simulink model "Regenerative_Brakes_PMSM_simscape"  (R2025b)
settings: Solver=ode23t  StartTime=0.0  StopTime=2.5  RelTol=1e-3  EnableMultiTasking=on
undefined symbols (not defined in the file): PermanentMagnetSynchrono_class, sigbuilder_block, Three_PhaseFault_class, UniversalBridge_class
libraries: nesl_utility x15, fl_lib x12, ee_lib x7, eeTransforms x2
settings Model: Creator=noname
settings SolverCC: AlgebraicLoopSolver=TrustRegion
settings DataIOCC: LimitDataPoints=on  SaveFormat=Array  ReturnWorkspaceOutputs=off
settings OptimizationCC: LifeSpan=inf
settings DebuggingCC: SaveWithParameterizedLinksMsg=none  UnderspecifiedInitializationDetection=Classic  MergeDetectMultiDrivingBlocksExec=none  SolverPrmCheckMsg=warning  UnconnectedInputMsg=warning  UnconnectedOutputMsg=warning  UnconnectedLineMsg=warning  StateNameClashWarn=warning  SFUnexpectedBacktrackingDiag=warning  SFNoUnconditionalDefaultTransitionDiag=warning  SFExecutionAtInitializationDiag=none  ArithmeticOperatorsInVariantConditions=warning
settings HardwareCC: ProdBitPerPointer=32.0  ProdBitPerSizeT=32.0  ProdBitPerPtrDiffT=32.0  ProdLargestAtomicFloat=None  ProdIntDivRoundTo=Undefined  ProdEndianess=Unspecified  ProdWordSize=32.0  ProdHWDeviceType=32-bit Generic
settings ModelReferenceCC: EnableRefExpFcnMdlSchedulingChecks=on  PropagateSignalLabelsOutOfModel=off
settings SFSimCC: SimUseLocalCustomCode=off  CustomCodeUndefinedFunction=UseInterfaceOnly
settings RTWCC: RTWUseLocalCustomCode=off  GPUComputeCapability=3.5  DLArmComputeVersion=19.05
settings CodeAppCC: StateflowObjectComments=on
settings GRTTargetCC: TargetLangStandard=C89/C90 (ANSI)
settings ConfigComp: CovMetricSettings=dw  CovSaveCumulativeToWorkspaceVar=on  CovSaveSingleToWorkspaceVar=on  CovExternalEMLEnable=off
settings SimscapeCC: SimscapeNormalizeSystem=off

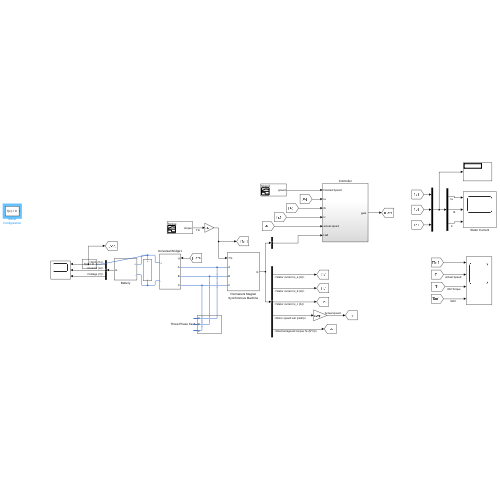
[thumbnail: Simulink's stored preview of the top-level diagram]
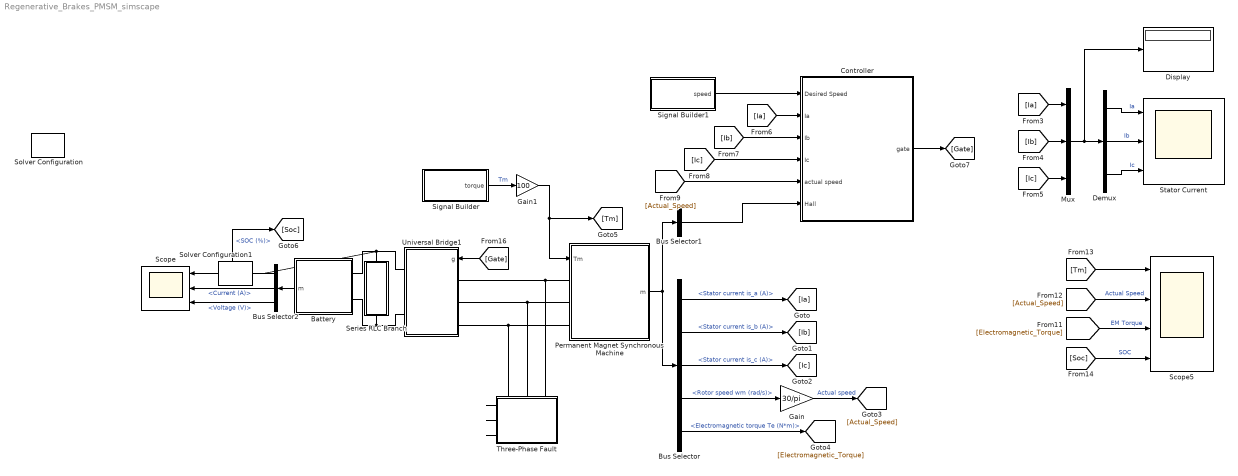
== system Regenerative_Brakes_PMSM_simscape ==
  Battery : Subsystem
      settings: OpenFcn=elec.conv.unmask(gcb);
  Bus Selector : BusSelector  OutputSignals=Stator current is_a (A),Stator current is_b (A),Stator current is_c (A),Rotor speed wm (rad/s),Electromagnetic torque Te (N*m)
  Bus Selector1 : BusSelector  OutputSignals=Hall effect signal h_a,Hall effect signal h_b,Hall effect signal h_c  OutputAsBus=on
  Bus Selector2 : BusSelector  OutputSignals=SOC (%),Current (A),Voltage (V)
  Controller : Subsystem
  Demux : Demux  Outputs=3
  Display : Display
  Gain : Gain  Gain=30/pi
  Gain1 : Gain  Gain=100
  Mux : Mux  Inputs=3
  Permanent Magnet Synchronous Machine : Subsystem
      settings: OpenFcn=elec.conv.unmask(gcb);
  Scope : Scope  NumInputPorts=3
      settings: ActiveDisplayYMinimum=79.5644  ActiveDisplayYMaximum=80.0484
  Scope5 : Scope  NumInputPorts=4
      settings: ActiveDisplayYMinimum=-400  ActiveDisplayYMaximum=600  DataLoggingVariableName=ScopeData13
  Series RLC Branch : Subsystem
      settings: OpenFcn=elec.conv.unmask(gcb);
  Signal Builder : Subsystem  Tag=STV Subsys  LoadFcn=sigbuilder_block('load');  StartFcn=sigbuilder_block('start');  StopFcn=sigbuilder_block('stop');  ClipboardFcn=sigbuilder_block('clipboard');  mask(Sigbuilder block){tuvar=[0:10]}
      mask help: Simulink:masks:SigbuilderBlock_MD
      mask init:
      | if ~strcmp(get_param(bdroot(gcbh),'SimulationStatus'),'stopped') tuvar = sigbuilder_block('maskInit'); end
      settings: CopyFcn=sigbuilder_block('copy');  DeleteFcn=sigbuilder_block('delete');  ModelCloseFcn=sigbuilder_block('modelClose');  PreSaveFcn=sigbuilder_block('preSave');  PauseFcn=sigbuilder_block('pause');  ContinueFcn=sigbuilder_block('continue');  NameChangeFcn=sigbuilder_block('namechange');  OpenFcn=sigbuilder_block('open',[437.25 183.75 550.5 395.25 ]);  CloseFcn=sigbuilder_block('close');
      mask Display: plot(0, 0, 100, 100,[2, 2, 32, 32, 2], [68, 8, 8, 68, 68],[32, 2], [38, 38], [32, 19, 2],[53, 60, 44], [32, 17, 17, 2],[16, 16, 31, 31]);txt = getActiveGroup(gcbh);text(2, 100, txt,'verticalAlignment', 'top');
  Signal Builder1 : Subsystem  Tag=STV Subsys  LoadFcn=sigbuilder_block('load');  StartFcn=sigbuilder_block('start');  StopFcn=sigbuilder_block('stop');  ClipboardFcn=sigbuilder_block('clipboard');  mask(Sigbuilder block){tuvar=[0:10]}
      mask help: Simulink:masks:SigbuilderBlock_MD
      mask init:
      | if ~strcmp(get_param(bdroot(gcbh),'SimulationStatus'),'stopped') tuvar = sigbuilder_block('maskInit'); end
      settings: CopyFcn=sigbuilder_block('copy');  DeleteFcn=sigbuilder_block('delete');  ModelCloseFcn=sigbuilder_block('modelClose');  PreSaveFcn=sigbuilder_block('preSave');  PauseFcn=sigbuilder_block('pause');  ContinueFcn=sigbuilder_block('continue');  NameChangeFcn=sigbuilder_block('namechange');  OpenFcn=sigbuilder_block('open',[6.75 6.75 1138.5 568.5 ]);  CloseFcn=sigbuilder_block('close');
      mask Display: plot(0, 0, 100, 100,[2, 2, 32, 32, 2], [68, 8, 8, 68, 68],[32, 2], [38, 38], [32, 19, 2],[53, 60, 44], [32, 17, 17, 2],[16, 16, 31, 31]);txt = getActiveGroup(gcbh);text(2, 100, txt,'verticalAlignment', 'top');
  Solver Configuration : nesl_utility/Solver Configuration  PhysicalDomain=network_engine_domain  SubClassName=solver  LeftPortType=input  RightPortType=generic  Tones=[]  Harmonics=[]  SimulateNoise=off  Profile=off  UseLocalSampling=off  EnableSwitchedLinearOptims=on  FrequencyDomain=off  UseCCode=off  RelTol=0.001  AbsTol=0.001  MinStep=1e-09  ToWorkspace=off  RevertToSquareIcSolve=off  NumHomotopyIterations=100  PhasorMode=off  PhasorModeNumHarmonics=1  ConsistencySolver=NEWTON_XTOL_AFTER_FTOL  IndexReductionMethod=DerivativeReplacement  DoDC=off  ResidualTolerance=1e-09  ConsistencyTolSource=GLOBAL  ConsistencyAbsTol=0.001  ConsistencyRelTol=0.001  ConsistencyTolFactor=0.001  UseLocalSolver=off  LocalSolverChoice=NE_BACKWARD_EULER_ADVANCER  ResolveIndetEquations=on  FunctionEvalNumThread=1  LocalSolverSampleTime=0.001  DoFixedCost=off  MaxNonlinIter=3  MaxModeIter=2  ComputeImpulses=off  ImpulseIterations=2  LinearAlgebra=auto  LinearAlgebraNumThread=0  EquationFormulation=NE_TIME_EF  DelaysMemoryBudget=1024  AutomaticFiltering=on  FilteringTimeConstant=0.001  PartitionStorageMethod=AS_NEEDED  PartitionMemoryBudget=1024  PartitionMethod=ROBUST  MultibodyUseLocalSolver=off  MultibodyLocalSolverChoice=ODE1  MultibodyLocalSolverSampleTime=0.001
  Solver Configuration1 : nesl_utility/Solver Configuration  PhysicalDomain=network_engine_domain  SubClassName=solver  LeftPortType=input  RightPortType=generic  Tones=[]  Harmonics=[]  SimulateNoise=off  Profile=off  UseLocalSampling=off  EnableSwitchedLinearOptims=on  FrequencyDomain=off  UseCCode=off  RelTol=0.001  AbsTol=0.001  MinStep=1e-09  ToWorkspace=off  RevertToSquareIcSolve=off  NumHomotopyIterations=100  PhasorMode=off  PhasorModeNumHarmonics=1  ConsistencySolver=NEWTON_XTOL_AFTER_FTOL  IndexReductionMethod=DerivativeReplacement  DoDC=off  ResidualTolerance=1e-09  ConsistencyTolSource=GLOBAL  ConsistencyAbsTol=0.001  ConsistencyRelTol=0.001  ConsistencyTolFactor=0.001  UseLocalSolver=off  LocalSolverChoice=NE_BACKWARD_EULER_ADVANCER  ResolveIndetEquations=on  FunctionEvalNumThread=1  LocalSolverSampleTime=0.001  DoFixedCost=off  MaxNonlinIter=3  MaxModeIter=2  ComputeImpulses=off  ImpulseIterations=2  LinearAlgebra=auto  LinearAlgebraNumThread=0  EquationFormulation=NE_TIME_EF  DelaysMemoryBudget=1024  AutomaticFiltering=on  FilteringTimeConstant=0.001  PartitionStorageMethod=AS_NEEDED  PartitionMemoryBudget=1024  PartitionMethod=ROBUST  MultibodyUseLocalSolver=off  MultibodyLocalSolverChoice=ODE1  MultibodyLocalSolverSampleTime=0.001
  Stator Current : Scope  NumInputPorts=3
      settings: ActiveDisplayYMinimum=-124.07803  ActiveDisplayYMaximum=125.94528
  Three-Phase Fault : Subsystem
      settings: OpenFcn=elec.conv.unmask(gcb);
  Universal Bridge1 : Subsystem
      settings: OpenFcn=elec.conv.unmask(gcb);
  wires:
  Permanent Magnet Synchronous Machine/1(m) -> Bus Selector/1, Bus Selector1/1
  Bus Selector/1 -> [Ia]  "<Stator current is_a (A)>"
  Bus Selector/2 -> [Ib]  "<Stator current is_b (A)>"
  Bus Selector/3 -> [Ic]  "<Stator current is_c (A)>"
  Bus Selector/4 -> Gain/1  "<Rotor speed wm (rad/s)>"
  Bus Selector1/1 -> Controller/6("Hall ")
  Gain/1 -> [Actual_Speed]  "Actual speed"
  Controller/1("gate ") -> [Gate]
  Battery/1(m) -> Bus Selector2/1
  Bus Selector2/1 -> Scope/1, [Soc]  "<SOC (%)>"
  Bus Selector2/2 -> Scope/2  "<Current (A)>"
  Bus Selector2/3 -> Scope/3  "<Voltage (V)>"
  Mux/1 -> Display/1, Demux/1
  Signal Builder/1(torque) -> Gain1/1  "Tm"
  Bus Selector/5 -> [Electromagnetic_Torque]  "<Electromagnetic torque Te (N*m)>"
  [Ia] -> Mux/1
  [Ib] -> Mux/2
  [Ic] -> Mux/3
  [Ia] -> Controller/2(Ia)
  [Ib] -> Controller/3(Ib)
  [Ic] -> Controller/4(Ic)
  [Actual_Speed] -> Controller/5(actual speed)
  [Actual_Speed] -> Scope5/2  "Actual Speed"
  [Tm] -> Scope5/1
  [Soc] -> Scope5/4  "SOC"
  [Gate] -> Universal Bridge1/1(g)
  Signal Builder1/1(speed) -> Controller/1(Desired Speed)
  Demux/1 -> Stator Current/1  "Ia"
  Demux/2 -> Stator Current/2  "Ib"
  Demux/3 -> Stator Current/3  "Ic"
  [Electromagnetic_Torque] -> Scope5/3  "EM Torque"
  Gain1/1 -> Permanent Magnet Synchronous Machine/1(Tm), [Tm]
  connections:
  Universal Bridge1/LConn1 -- Three-Phase Fault/LConn1 -- Permanent Magnet Synchronous Machine/LConn1
  Permanent Magnet Synchronous Machine/LConn2 -- Universal Bridge1/LConn2 -- Three-Phase Fault/LConn2
  Universal Bridge1/LConn3 -- Three-Phase Fault/LConn3 -- Permanent Magnet Synchronous Machine/LConn3
  Series RLC Branch/LConn1 -- Universal Bridge1/RConn1 -- Battery/LConn1 -- Solver Configuration1/RConn1
  Series RLC Branch/RConn1 -- Battery/LConn2 -- Universal Bridge1/RConn2

== system Regenerative_Brakes_PMSM_simscape/Battery ==
  + : PMIOPort  Side=Left
  - : PMIOPort  Port=2  Side=Left
  m : Outport  VectorParamsAs1DForOutWhenUnconnected=off

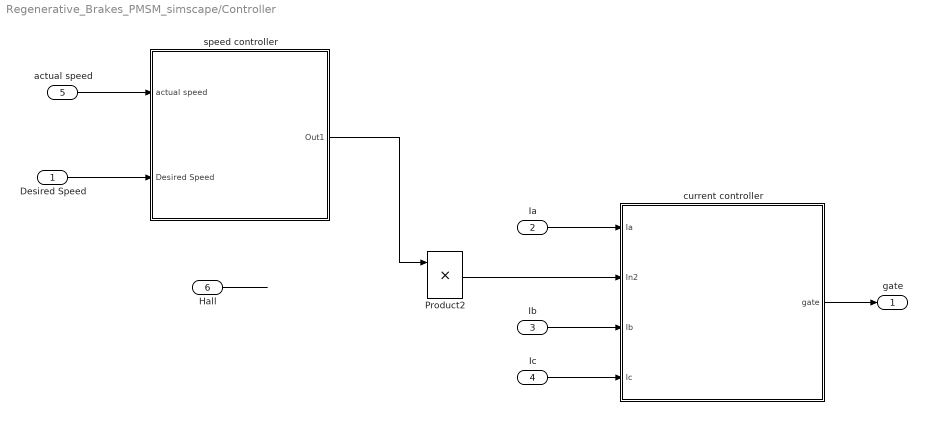
== system Regenerative_Brakes_PMSM_simscape/Controller ==
  Desired Speed : Inport
  Ia : Inport  Port=2
  Ib : Inport  Port=3
  Ic : Inport  Port=4
  actual speed : Inport  Port=5
  "Hall " : Inport  Port=6
  Product2 : Product  SaturateOnIntegerOverflow=on  OutDataTypeStr=Inherit: Same as first input
  current controller : Subsystem
  speed controller : Subsystem
  "gate " : Outport  VectorParamsAs1DForOutWhenUnconnected=off
  wires:
  "Hall "/1 -> ?
  ? -> Product2/2
  current controller/1("gate ") -> "gate "/1
  Ic/1 -> current controller/4(Ic)
  Ib/1 -> current controller/3(Ib)
  Ia/1 -> current controller/1(Ia)
  Product2/1 -> current controller/2(In2)
  actual speed/1 -> speed controller/1(actual speed)
  speed controller/1(Out1) -> Product2/1
  Desired Speed/1 -> speed controller/2(Desired Speed)

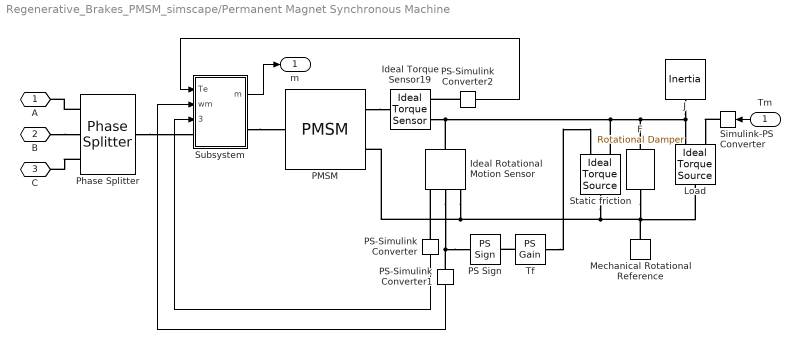
== system Regenerative_Brakes_PMSM_simscape/Permanent Magnet Synchronous Machine ==
  Tm : Inport
  F : fl_lib/Mechanical/Rotational Elements/Rotational Damper  D=0.000425 N*m/(rad/s)  w_specify=on  w_priority=High  w=0 rad/s  w_nominal_specify=off  w_nominal_value=1  w_nominal_unit=rad/s  t_specify=off  t_priority=None  t=0 N*m  t_nominal_specify=off  t_nominal_value=1  t_nominal_unit=N*m
  Ideal Rotational Motion Sensor : fl_lib/Mechanical/Mechanical Sensors/Ideal Rotational Motion Sensor  reference=foundation.enum.MeasurementReference.difference  acceleration_port=false  velocity_port=true  position_port=true  wrap_angle=simscape.enum.onoff.off  offset=0 deg
  Ideal Torque Sensor19 : fl_lib/Mechanical/Mechanical Sensors/Ideal Torque Sensor
  J : fl_lib/Mechanical/Rotational Elements/Inertia  inertia=0.003334 kg*m^2  num_ports=foundation.enum.numPorts2.one  w_specify=on  w_priority=High  w=0 rad/s  w_nominal_specify=off  w_nominal_value=1  w_nominal_unit=rad/s  t_specify=off  t_priority=None  t=0 N*m  t_nominal_specify=off  t_nominal_value=1  t_nominal_unit=N*m
  Load : fl_lib/Mechanical/Mechanical Sources/Ideal Torque Source
  Mechanical Rotational Reference : fl_lib/Mechanical/Rotational Elements/Mechanical Rotational Reference
  PMSM : ee_lib/Electromechanical/Permanent Magnet/PMSM  port_option=ee.enum.threePhasePort.composite  winding_type=ee.enum.statorconnection.wye  machine_param=ee.enum.pmsm.parameterization.constant  nPolePairs=4  pmflux_param=1  pm_flux_linkage=PermanentMagnetSynchrono_class('Torque Tm',[0.003334 0.000425 4 0],4,'Flux linkage established by magnets (V.s)',0.1821,132.1171,1.0926,'90 degrees behind phase A axis (modified Park)',[0 0 0 0],'Sinusoidal',120,'3',[0 0 0 0 0 0]).objParamMappingDerived.NewDerivedParam.pm_flux_linkage Wb  torque_constant=0.18 N*m/A  back_emf_constant=0.18 V/(rad/s)  stator_param=1  Ld=0.00153 H  Lq=0.00153 H  idVec=[-200, 0, 200] A  iqVec=[-200, 0, 200] A  LdMatrix=0.0002 * ones(3, 3) H  LqMatrix=0.0002 * ones(3, 3) H  PmMatrix=0.1 * ones(3, 3) Wb  ktMatrix=0.18 * ones(3, 3) N*m/A  keMatrix=0.18 * ones(3, 3) V/(rad/s)  L0=1e-09 H  Ls=0.0002 H  Lm=-0.00002 H  Ms=0.00002 H  Rs=0.129 Ohm  zero_sequence=0  axes_param=1  loss_param=ee.enum.ironloss.none  losses_oc=[0, 0, 0] W  losses_sc=[0, 0, 0] W  f_losses=60 Hz  Isc_losses=95 A  J=0 kg*m^2  lam=0 N*m/(rad/s)  i_d_specify=on  i_d_priority=High  i_d=PermanentMagnetSynchrono_class('Torque Tm',[0.003334 0.000425 4 0],4,'Flux linkage established by magnets (V.s)',0.1821,132.1171,1.0926,'90 degrees behind phase A axis (modified Park)',[0 0 0 0],'Sinusoidal',120,'3',[0 0 0 0 0 0]).objParamMappingDerived.NewDerivedParam.i_d A  i_d_nominal_specify=off  i_d_nominal_value=1  i_d_nominal_unit=A  i_q_specify=on  i_q_priority=High  i_q=PermanentMagnetSynchrono_class('Torque Tm',[0.003334 0.000425 4 0],4,'Flux linkage established by magnets (V.s)',0.1821,132.1171,1.0926,'90 degrees behind phase A axis (modified Park)',[0 0 0 0],'Sinusoidal',120,'3',[0 0 0 0 0 0]).objParamMappingDerived.NewDerivedParam.i_q A  i_q_nominal_specify=off  i_q_nominal_value=1  i_q_nominal_unit=A  torque_specify=off  torque_priority=None  torque=0 N*m  torque_nominal_specify=off  torque_nominal_value=1  torque_nominal_unit=N*m  angular_velocity_specify=on  angular_velocity_priority=High  angular_velocity=0 rad/s  angular_velocity_nominal_specify=off  angular_velocity_nominal_value=1  angular_velocity_nominal_unit=rpm  angular_position_specify=on  angular_position_priority=High  angular_position=0 deg  angular_position_nominal_specify=off  angular_position_nominal_value=1  angular_position_nominal_unit=deg  alpha=3.93e-3 1/K  alpha_flux=-0.001 1/K  Tmeas=298.15 K  stator_thermal_mass=100 J/K  rotor_thermal_mass=200 J/K  Rm_percent_rotor=90  Rd_percent_rotor=30  temperatureA_specify=off  temperatureA_priority=High  temperatureA=25 degC  temperatureA_nominal_specify=off  temperatureA_nominal_value=1  temperatureA_nominal_unit=degC  temperatureB_specify=off  temperatureB_priority=High  temperatureB=25 degC  temperatureB_nominal_specify=off  temperatureB_nominal_value=1  temperatureB_nominal_unit=degC  temperatureC_specify=off  temperatureC_priority=High  temperatureC=25 degC  temperatureC_nominal_specify=off  temperatureC_nominal_value=1  temperatureC_nominal_unit=degC  temperatureR_specify=off  temperatureR_priority=High  temperatureR=25 degC  temperatureR_nominal_specify=off  temperatureR_nominal_value=1  temperatureR_nominal_unit=degC
      settings: InternalSimscapePortConfiguration="{\"Bottom\":[],\"Left\":[{\"id\":\"N\",\"label\":\"~\",\"type\":\"foundation.electrical.three_phase\"}],\"Right\":[{\"id\":\"R\",\"label\":\"R\",\"type\":\"foundation.mechanical.rotational.rotational\"},{\"id\":\"C\",\"label\":\"C\",\"type\":\"foundation.mechanical.rotational.rotational\"}],\"Top\":[]}"
  PS Sign : fl_lib/Physical Signals/Nonlinear Operators/PS Sign
      settings: InternalSimscapePortConfiguration="{\"Bottom\":[],\"Left\":[{\"id\":\"I\",\"label\":\"\",\"type\":\"input\"}],\"Right\":[{\"id\":\"O\",\"label\":\"\",\"type\":\"output\"}],\"Top\":[]}"
  PS-Simulink Converter : nesl_utility/PS-Simulink Converter  PhysicalDomain=network_engine_domain  SubClassName=ps_output  LeftPortType=input  RightPortType=output  PseudoPeriodic=off  Frequencies=[]  VectorFormat=1-D array  Unit=1  AffineConversion=off
  PS-Simulink Converter1 : nesl_utility/PS-Simulink Converter  PhysicalDomain=network_engine_domain  SubClassName=ps_output  LeftPortType=input  RightPortType=output  PseudoPeriodic=off  Frequencies=[]  VectorFormat=1-D array  Unit=1  AffineConversion=off
  PS-Simulink Converter2 : nesl_utility/PS-Simulink Converter  PhysicalDomain=network_engine_domain  SubClassName=ps_output  LeftPortType=input  RightPortType=output  PseudoPeriodic=off  Frequencies=[]  VectorFormat=1-D array  Unit=1  AffineConversion=off
  Phase Splitter : ee_lib/Connectors & References/Phase Splitter
  Simulink-PS Converter : nesl_utility/Simulink-PS Converter  PhysicalDomain=network_engine_domain  SubClassName=ps_input  LeftPortType=input  RightPortType=output  PseudoPeriodic=off  Frequencies=[]  NoiseDistribution=none  NoiseParameters=[]  Unit=1  AffineConversion=off  FilteringAndDerivatives=provide  SimscapeFilterOrder=1  InputFilterTimeConstant=0.001  UdotUserProvided=0
  Static friction : fl_lib/Mechanical/Mechanical Sources/Ideal Torque Source
  Subsystem : Subsystem
  Tf : fl_lib/Physical Signals/Functions/PS Gain  gain=PermanentMagnetSynchrono_class('Torque Tm',[0.003334 0.000425 4 0],4,'Flux linkage established by magnets (V.s)',0.1821,132.1171,1.0926,'90 degrees behind phase A axis (modified Park)',[0 0 0 0],'Sinusoidal',120,'3',[0 0 0 0 0 0]).objParamMappingDerived.NewDerivedParam.Tf
  A : PMIOPort  Side=Left
  B : PMIOPort  Port=2  Side=Left
  C : PMIOPort  Port=3  Side=Left
  m : Outport  VectorParamsAs1DForOutWhenUnconnected=off
  wires:
  PS-Simulink Converter1/1 -> Subsystem/2(wm)
  PS-Simulink Converter/1 -> Subsystem/3(thetam)
  PS-Simulink Converter2/1 -> Subsystem/1(Te)
  Subsystem/1(m) -> m/1
  Tm/1 -> Simulink-PS Converter/1
  connections:
  PS-Simulink Converter2/LConn1 -- Ideal Torque Sensor19/RConn2
  Phase Splitter/LConn1 -- Subsystem/LConn1
  Subsystem/RConn1 -- PMSM/LConn1
  PS-Simulink Converter/LConn1 -- Ideal Rotational Motion Sensor/RConn3
  Tf/RConn1 -- Static friction/RConn1
  PS Sign/LConn1 -- PS-Simulink Converter1/LConn1 -- Ideal Rotational Motion Sensor/RConn2
  Tf/LConn1 -- PS Sign/RConn1
  PMSM/RConn1 -- Ideal Torque Sensor19/LConn1
  Ideal Torque Sensor19/RConn1 -- Static friction/RConn2 -- F/LConn1 -- Load/RConn2 -- J/LConn1 -- Ideal Rotational Motion Sensor/LConn1
  Phase Splitter/RConn3 -- C/RConn1
  Phase Splitter/RConn1 -- A/RConn1
  B/RConn1 -- Phase Splitter/RConn2
  Simulink-PS Converter/RConn1 -- Load/RConn1
  Load/LConn1 -- F/RConn1 -- Static friction/LConn1 -- PMSM/RConn2 -- Ideal Rotational Motion Sensor/RConn1 -- Mechanical Rotational Reference/LConn1

== system Regenerative_Brakes_PMSM_simscape/Series RLC Branch ==
  Capacitor : fl_lib/Electrical/Electrical Elements/Capacitor  c=0.075 F  r=1e-6 Ohm  g=0 1/Ohm  i_specify=off  i_priority=None  i=0 A  i_nominal_specify=off  i_nominal_value=1  i_nominal_unit=A  v_specify=off  v_priority=None  v=0 V  v_nominal_specify=off  v_nominal_value=1  v_nominal_unit=V  vc_specify=on  vc_priority=None  vc=0 V  vc_nominal_specify=off  vc_nominal_value=1  vc_nominal_unit=V
  + : PMIOPort  Side=Left
  - : PMIOPort  Port=2  Side=Right
  connections:
  Capacitor/RConn1 -- -/RConn1
  +/RConn1 -- Capacitor/LConn1

== system Regenerative_Brakes_PMSM_simscape/Signal Builder ==
  Demux : Demux  Tag=STV Demux  Outputs=1
      settings: DisplayOption=none
  FromWs : FromWorkspace  Tag=STV FromWs  VariableName=tuvar
      SigBuilderData=|
      | common.afterFinalStr = 'Extrapolate'
      | common.sampleTime = 0
      | dataSet.timeRange = [0 2.5]
      | dataSet.name = 'Torque'
      | sbobj.Name = 'Signal Builder'
      | sbobj.Groups.Name = 'Torque'
      | sbobj.Groups.Signals.Name = 'torque'
      | sbobj.Groups.Signals.XData = [0 0.05 0.05 0.5 0.5 0.75 0.75 1.25 1.25 1.65 1.65 2.05 2.05 2.35 2.35 2.5]
      | sbobj.Groups.Signals.YData = [0 0 5 5 -1 -1 -3 -3 1.5 1.5 5 5 4 4 -1 -1]
      | sbobj.Groups.TimeRange = [0 2.5]
  torque : Outport  VectorParamsAs1DForOutWhenUnconnected=off
  wires:
  Demux/1 -> torque/1
  FromWs/1 -> Demux/1

== system Regenerative_Brakes_PMSM_simscape/Signal Builder1 ==
  Demux : Demux  Tag=STV Demux  Outputs=1
      settings: DisplayOption=none
  FromWs : FromWorkspace  Tag=STV FromWs  VariableName=tuvar
      SigBuilderData=|
      | common.afterFinalStr = 'Extrapolate'
      | common.sampleTime = 0
      | dataSet.timeRange = [0 2.5]
      | dataSet.name = 'Speed'
      | sbobj.Name = 'Signal Builder'
      | sbobj.Groups.Name = 'Speed'
      | sbobj.Groups.Signals.Name = 'speed'
      | sbobj.Groups.Signals.XData = [0 0.05 0.5 0.75 1 1.5 2 2.35 2.5]
      | sbobj.Groups.Signals.YData = [0 0 2500 2500 1000 1000 2000 2000 1000]
      | sbobj.Groups.TimeRange = [0 2.5]
  speed : Outport  VectorParamsAs1DForOutWhenUnconnected=off
  wires:
  Demux/1 -> speed/1
  FromWs/1 -> Demux/1

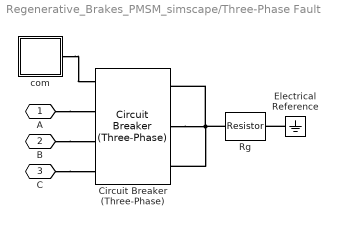
== system Regenerative_Brakes_PMSM_simscape/Three-Phase Fault ==
  Circuit Breaker (Three-Phase) : ee_lib/Switches & Breakers/Circuit Breaker (Three-Phase)  R_closed=0.001 Ohm  G_open=Three_PhaseFault_class(0,[0.0166666666666667 0.0833333333333333],NaN,0.01,1000000,Inf,'on','off').objParamMappingDerived.NewDerivedParam.G_open 1/Ohm  threshold=0.5 V  breaker_behavior=ee.enum.switches.breakerBehavior.zeroCrossingEnable
      settings: InternalSimscapePortConfiguration="{\"Bottom\":[],\"Left\":[{\"id\":\"vT\",\"label\":\"vT\",\"type\":\"input\"},{\"id\":\"a1\",\"label\":\"a1\",\"type\":\"foundation.electrical.electrical\"},{\"id\":\"b1\",\"label\":\"b1\",\"type\":\"foundation.electrical.electrical\"},{\"id\":\"c1\",\"label\":\"c1\",\"type\":\"foundation.electrical.electrical\"}],\"Right\":[{\"id\":\"a2\",\"label\":\"a2\",\"type\":\"foundation.electrical.electrical\"},{\"id\":\"b2\",\"label\":\"b2\",\"type\":\"foundation.electrical.electrical\"},{\"id\":\"c2\",\"label\":\"c2\",\"type\":\"foundation.electrical.electrical\"}],\"Top\":[]}"
  Electrical Reference : fl_lib/Electrical/Electrical Elements/Electrical Reference
  Rg : fl_lib/Electrical/Electrical Elements/Resistor  R=Three_PhaseFault_class(0,[0.0166666666666667 0.0833333333333333],NaN,0.01,1000000,Inf,'on','off').objParamMappingDerived.NewDerivedParam.R_ng_fault Ohm  i_specify=off  i_priority=None  i=0 A  i_nominal_specify=off  i_nominal_value=1  i_nominal_unit=A  v_specify=off  v_priority=None  v=0 V  v_nominal_specify=off  v_nominal_value=1  v_nominal_unit=V
  com : Subsystem
  A : PMIOPort  Side=Left
  B : PMIOPort  Port=2  Side=Left
  C : PMIOPort  Port=3  Side=Left
  connections:
  com/RConn1 -- Circuit Breaker (Three-Phase)/LConn1
  Electrical Reference/LConn1 -- Rg/RConn1
  Rg/LConn1 -- Circuit Breaker (Three-Phase)/RConn1 -- Circuit Breaker (Three-Phase)/RConn2 -- Circuit Breaker (Three-Phase)/RConn3
  A/RConn1 -- Circuit Breaker (Three-Phase)/LConn2
  B/RConn1 -- Circuit Breaker (Three-Phase)/LConn3
  C/RConn1 -- Circuit Breaker (Three-Phase)/LConn4

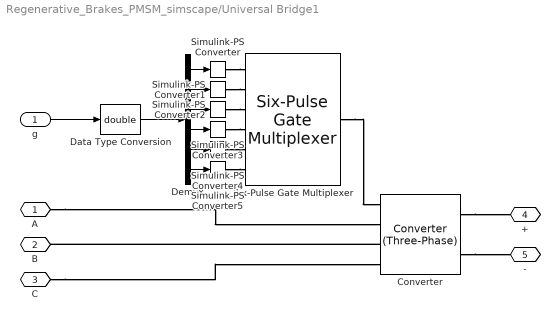
== system Regenerative_Brakes_PMSM_simscape/Universal Bridge1 ==
  g : Inport
  Converter : ee_lib/Semiconductors & Converters/Converters/Converter (Three-Phase)  port_option=ee.enum.threePhasePort.expanded  fidelity_option=ee.enum.converters.fidelity.detailed  device_type=4  showThermalPort=false  K=0  Vth=0.5 V  Vgt=0.5 V  Vgt_off=0.1 V  Ih=0.1 A  Vf=UniversalBridge_class('3','MOSFET / Diodes',[0 0],0,100000,Inf,0.001).objParamMappingDerived.NewDerivedParam.Vf V  Ron=UniversalBridge_class('3','MOSFET / Diodes',[0 0],0,100000,Inf,0.001).objParamMappingDerived.NewDerivedParam.Ron Ohm  Rds=UniversalBridge_class('3','MOSFET / Diodes',[0 0],0,100000,Inf,0.001).objParamMappingDerived.NewDerivedParam.Rds Ohm  Goff=UniversalBridge_class('3','MOSFET / Diodes',[0 0],0,100000,Inf,0.001).objParamMappingDerived.NewDerivedParam.Goff 1/Ohm  Eon_scalar=22.86e-3 J  Eoff_scalar=17.14e-3 J  Eoff_natural_commutation=10e-3 J  Voff=300 V  Iout_scalar=600 A  onCurrentMeasDelay=0 s  useCurrentFromPreviousCycle=false  useVoltageFromPreviousCycle=false  diode_param=2  diode_Vf=UniversalBridge_class('3','MOSFET / Diodes',[0 0],0,100000,Inf,0.001).objParamMappingDerived.NewDerivedParam.diode_Vf V  diode_Ron=UniversalBridge_class('3','MOSFET / Diodes',[0 0],0,100000,Inf,0.001).objParamMappingDerived.NewDerivedParam.diode_Ron Ohm  diode_Goff=UniversalBridge_class('3','MOSFET / Diodes',[0 0],0,100000,Inf,0.001).objParamMappingDerived.NewDerivedParam.diode_Goff 1/Ohm  diode_C=50 nF  diode_iRM=-235 A  diode_iF=300 A  diode_idot=-50 A/us  diode_trr_param=ee.enum.converters.diodetrr.trr_factor  diode_trr_factor=3  diode_trr=15 us  diode_Qrr=1.5e+3 s*uA  diode_rec_loss_model=ee.enum.diode.reverseRecoveryModel.fixed  diode_ErecVal=0 J  diode_scaleWithIandV=false  diode_ErecMat=zeros(2, 3) J  diode_TjrecVec=[298.15, 398.15] K  diode_IfrecVec=[.1, 1, 10] A  diode_IrecVal=10 A  diode_VrecVal=10 V  diode_tFilter=1 / 1000 / 100 s  thermal_network_parameterization=ee.enum.thermalNetworkTopology.external  Rth=[.08, .5] K/W  Rth_Cauer=[.08, .1, .5] K/W  Rth_Foster=[.08, .14, .22, .16] K/W  thermal_mass_parameterization=ee.enum.thermalNetwork.timeconstant  thermal_mass=[.01, .5] J/K  thermal_mass_Cauer=[.01, .1, .5] J/K  thermal_mass_Foster=[.001, .005, .05, .5] J/K  thermal_time_constant=[.001, .2] s  thermal_time_constant_Cauer=[.001, .1, .2] s  thermal_time_constant_Foster=[7e-05, .0007, .01, .08] s  thermal_mass_initial_temperatures=[25, 25] degC  thermal_mass_initial_temperatures_Cauer=[25, 25, 25] degC  junction_thermal_mass=0.01 J/K  Tvec_initial_Foster=[25, 25, 25, 25] degC  snubber_type=0  Cs=UniversalBridge_class('3','MOSFET / Diodes',[0 0],0,100000,Inf,0.001).objParamMappingDerived.NewDerivedParam.Cs F  Rs=UniversalBridge_class('3','MOSFET / Diodes',[0 0],0,100000,Inf,0.001).objParamMappingDerived.NewDerivedParam.Rs Ohm  Vce_loss=[0, 150, 300] V
      settings: InternalSimscapePortConfiguration="{\"Bottom\":[],\"Left\":[{\"id\":\"G\",\"label\":\"G\",\"type\":\"foundation.electrical.twelve_phase\"},{\"id\":\"a\",\"label\":\"a\",\"type\":\"foundation.electrical.electrical\"},{\"id\":\"b\",\"label\":\"b\",\"type\":\"foundation.electrical.electrical\"},{\"id\":\"c\",\"label\":\"c\",\"type\":\"foundation.electrical.electrical\"}],\"Right\":[{\"id\":\"p\",\"label\":\"+\",\"type\":\"foundation.electrical.electrical\"},{\"id\":\"n\",\"label\":\"-\",\"type\":\"foundation.electrical.electrical\"}],\"Top\":[]}"
  Data Type Conversion : DataTypeConversion  OutDataTypeStr=double  SaturateOnIntegerOverflow=off  RndMeth=Floor
  Demux : Demux  Outputs=6
  Simulink-PS Converter{,1..5} (6 alike) : nesl_utility/Simulink-PS Converter  PhysicalDomain=network_engine_domain  SubClassName=ps_input  LeftPortType=input  RightPortType=output  PseudoPeriodic=off  Frequencies=[]  NoiseDistribution=none  NoiseParameters=[]  Unit=1  AffineConversion=off  FilteringAndDerivatives=provide  SimscapeFilterOrder=1  InputFilterTimeConstant=0.001  UdotUserProvided=0
  Six-Pulse Gate Multiplexer : ee_lib/Semiconductors & Converters/Converters/Six-Pulse Gate Multiplexer  port_option=ee.enum.controlport.ps
  A : PMIOPort  Side=Left
  B : PMIOPort  Port=2  Side=Left
  C : PMIOPort  Port=3  Side=Left
  + : PMIOPort  Port=4  Side=Right
  - : PMIOPort  Port=5  Side=Right
  wires:
  Data Type Conversion/1 -> Demux/1
  Demux/6 -> Simulink-PS Converter5/1
  Demux/5 -> Simulink-PS Converter4/1
  Demux/4 -> Simulink-PS Converter3/1
  Demux/3 -> Simulink-PS Converter2/1
  Demux/2 -> Simulink-PS Converter1/1
  Demux/1 -> Simulink-PS Converter/1
  g/1 -> Data Type Conversion/1
  connections:
  Converter/RConn2 -- -/RConn1
  Converter/RConn1 -- +/RConn1
  C/RConn1 -- Converter/LConn4
  A/RConn1 -- Converter/LConn2
  Converter/LConn3 -- B/RConn1
  Simulink-PS Converter5/RConn1 -- Six-Pulse Gate Multiplexer/LConn6
  Simulink-PS Converter4/RConn1 -- Six-Pulse Gate Multiplexer/LConn5
  Simulink-PS Converter3/RConn1 -- Six-Pulse Gate Multiplexer/LConn4
  Simulink-PS Converter2/RConn1 -- Six-Pulse Gate Multiplexer/LConn3
  Simulink-PS Converter/RConn1 -- Six-Pulse Gate Multiplexer/LConn1
  Simulink-PS Converter1/RConn1 -- Six-Pulse Gate Multiplexer/LConn2
  Six-Pulse Gate Multiplexer/RConn1 -- Converter/LConn1

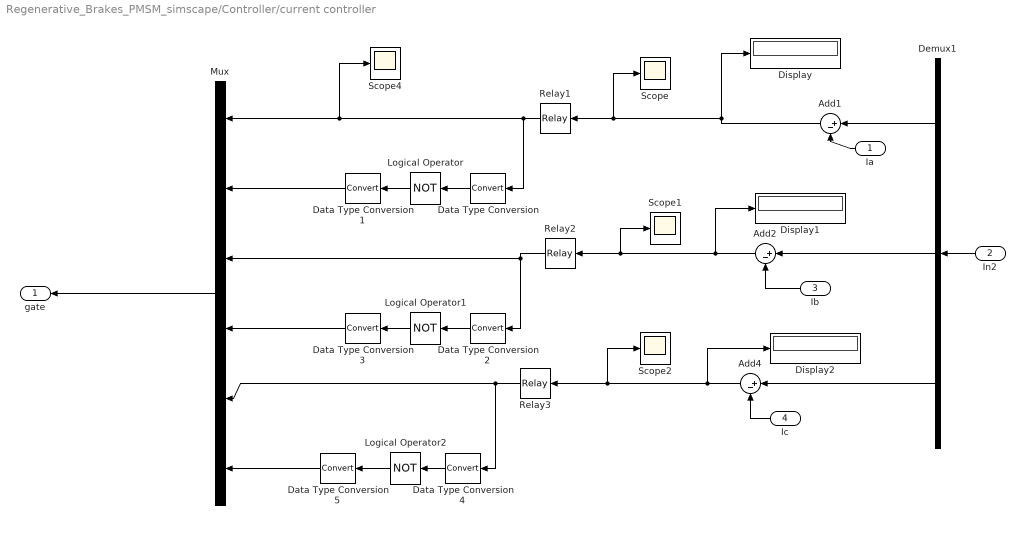
== system Regenerative_Brakes_PMSM_simscape/Controller/current controller ==
  Ia : Inport
  In2 : Inport  Port=2
  Ib : Inport  Port=3
  Ic : Inport  Port=4
  Add1 : Sum  Inputs=|+-
  Add2 : Sum  Inputs=|+-
  Add4 : Sum  Inputs=|+-
  Data Type Conversion{,1..5} (6 alike) : DataTypeConversion
  Demux1 : Demux  Outputs=3
      settings: DisplayOption=none
  Display : Display
  Display1 : Display
  Display2 : Display
  Logical Operator : Logic  Operator=NOT  AllPortsSameDT=off  OutDataTypeStr=boolean
  Logical Operator1 : Logic  Operator=NOT  AllPortsSameDT=off  OutDataTypeStr=boolean
  Logical Operator2 : Logic  Operator=NOT  AllPortsSameDT=off  OutDataTypeStr=boolean
  Mux : Mux  Inputs=6
  Relay1 : Relay  OnSwitchValue=5  OffSwitchValue=-5
  Relay2 : Relay  OnSwitchValue=5  OffSwitchValue=-5
  Relay3 : Relay  OnSwitchValue=5  OffSwitchValue=-5
  Scope{,1..2,4} (4 alike) : Scope
      Scope settings: DataLoggingVariableName=ScopeData6
      Scope1 settings: DataLoggingVariableName=ScopeData7
      Scope2 settings: DataLoggingVariableName=ScopeData8
      Scope4 settings: DataLoggingVariableName=ScopeData12
  "gate " : Outport  VectorParamsAs1DForOutWhenUnconnected=off
  wires:
  Relay1/1 -> Scope4/1, Mux/1, Data Type Conversion/1
  Relay2/1 -> Mux/3, Data Type Conversion2/1
  Relay3/1 -> Mux/5, Data Type Conversion4/1
  Ib/1 -> Add2/2
  Mux/1 -> "gate "/1
  Ic/1 -> Add4/2
  Add4/1 -> Display2/1, Scope2/1, Relay3/1
  Add2/1 -> Relay2/1, Scope1/1, Display1/1
  Add1/1 -> Display/1, Scope/1, Relay1/1
  Data Type Conversion/1 -> Logical Operator/1
  Logical Operator/1 -> Data Type Conversion1/1
  Data Type Conversion1/1 -> Mux/2
  Logical Operator1/1 -> Data Type Conversion3/1
  Data Type Conversion3/1 -> Mux/4
  Data Type Conversion2/1 -> Logical Operator1/1
  Data Type Conversion5/1 -> Mux/6
  Logical Operator2/1 -> Data Type Conversion5/1
  Data Type Conversion4/1 -> Logical Operator2/1
  Demux1/2 -> Add2/1
  Demux1/3 -> Add4/1
  In2/1 -> Demux1/1
  Ia/1 -> Add1/2
  Demux1/1 -> Add1/1

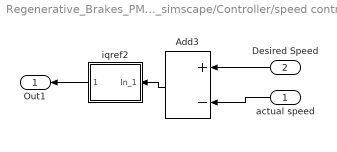
== system Regenerative_Brakes_PMSM_simscape/Controller/speed controller ==
  actual speed : Inport
  Desired Speed : Inport  Port=2
  Add3 : Sum  Inputs=+-
  iqref2 : Subsystem  mask(PI Controller){I=2.8, P=5, sat=[-inf, inf]}
      mask prompts: I "Integral"; P "Proportional:"; sat "Minimum and maximum outputs:"
      mask init:
      | min=sat(1);max=sat(2);
      mask Display: disp('PI')
  Out1 : Outport  VectorParamsAs1DForOutWhenUnconnected=off
  wires:
  actual speed/1 -> Add3/2
  Desired Speed/1 -> Add3/1
  Add3/1 -> iqref2/1(In_1)
  iqref2/1(Out_1) -> Out1/1

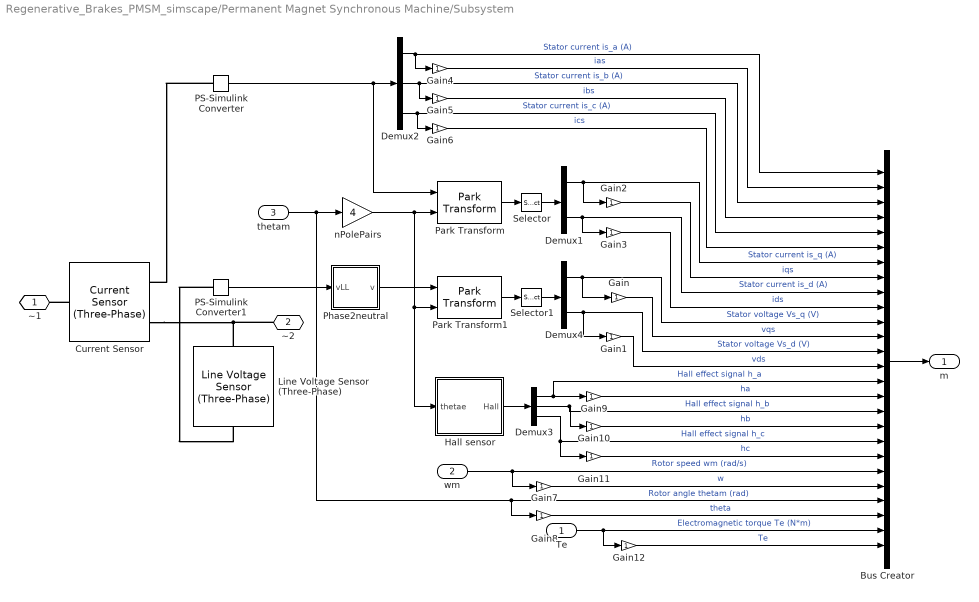
== system Regenerative_Brakes_PMSM_simscape/Permanent Magnet Synchronous Machine/Subsystem ==
  Te : Inport
  wm : Inport  Port=2
  thetam : Inport  Port=3
  Bus Creator : BusCreator  Inputs=26
  Current Sensor : ee_lib/Sensors & Transducers/Current Sensor (Three-Phase)
  Demux1 : Demux  Outputs=2
  Demux2 : Demux  Outputs=3
  Demux3 : Demux  Outputs=3
  Demux4 : Demux  Outputs=2
  Gain{,1..12} (13 alike) : Gain
  Hall sensor : Subsystem
  Line Voltage Sensor (Three-Phase) : ee_lib/Sensors & Transducers/Line Voltage Sensor (Three-Phase)
  PS-Simulink Converter : nesl_utility/PS-Simulink Converter  PhysicalDomain=network_engine_domain  SubClassName=ps_output  LeftPortType=input  RightPortType=output  PseudoPeriodic=off  Frequencies=[]  VectorFormat=1-D array  Unit=1  AffineConversion=off
  PS-Simulink Converter1 : nesl_utility/PS-Simulink Converter  PhysicalDomain=network_engine_domain  SubClassName=ps_output  LeftPortType=input  RightPortType=output  PseudoPeriodic=off  Frequencies=[]  VectorFormat=1-D array  Unit=1  AffineConversion=off
  Park Transform : eeTransforms/Park Transform  AxisAlignment=Q-axis  PowerInvariant=off
  Park Transform1 : eeTransforms/Park Transform  AxisAlignment=Q-axis  PowerInvariant=off
  Phase2neutral : Subsystem
  Selector : Selector  InputPortWidth=3  IndexOptions=Index vector (dialog)  Indices=[2 1]  OutputSizes=1
  Selector1 : Selector  InputPortWidth=3  IndexOptions=Index vector (dialog)  Indices=[2 1]  OutputSizes=1
  nPolePairs : Gain  Gain=4
  ~1 : PMIOPort  Side=Left
  ~2 : PMIOPort  Port=2  Side=Right
  m : Outport  VectorParamsAs1DForOutWhenUnconnected=off
  wires:
  Phase2neutral/1(v) -> Park Transform1/1
  Gain8/1 -> Bus Creator/24  "theta"
  Gain7/1 -> Bus Creator/22  "w"
  Selector1/1 -> Demux4/1
  Selector/1 -> Demux1/1
  Gain11/1 -> Bus Creator/20  "hc"
  Gain10/1 -> Bus Creator/18  "hb"
  Gain9/1 -> Bus Creator/16  "ha"
  Gain1/1 -> Bus Creator/14  "vds"
  Gain/1 -> Bus Creator/12  "vqs"
  Gain3/1 -> Bus Creator/10  "ids"
  Gain2/1 -> Bus Creator/8  "iqs"
  Hall sensor/1(Hall) -> Demux3/1
  PS-Simulink Converter1/1 -> Phase2neutral/1(vLL)
  Gain6/1 -> Bus Creator/6  "ics"
  Gain5/1 -> Bus Creator/4  "ibs"
  Gain4/1 -> Bus Creator/2  "ias"
  PS-Simulink Converter/1 -> Demux2/1, Park Transform/1
  Te/1 -> Bus Creator/25, Gain12/1  "Electromagnetic torque Te (N*m)"
  Gain12/1 -> Bus Creator/26  "Te"
  Demux3/3 -> Bus Creator/19, Gain11/1  "Hall effect signal h_c"
  Demux3/2 -> Gain10/1, Bus Creator/17  "Hall effect signal h_b"
  Demux3/1 -> Gain9/1, Bus Creator/15  "Hall effect signal h_a"
  thetam/1 -> nPolePairs/1, Gain8/1, Bus Creator/23  "Rotor angle thetam (rad)"
  Bus Creator/1 -> m/1
  Demux2/3 -> Bus Creator/5, Gain6/1  "Stator current is_c (A)"
  Demux2/2 -> Gain5/1, Bus Creator/3  "Stator current is_b (A)"
  Demux2/1 -> Gain4/1, Bus Creator/1  "Stator current is_a (A)"
  Demux1/2 -> Gain3/1, Bus Creator/9  "Stator current is_d (A)"
  Park Transform/1 -> Selector/1
  Demux1/1 -> Gain2/1, Bus Creator/7  "Stator current is_q (A)"
  Demux4/2 -> Gain1/1, Bus Creator/13  "Stator voltage Vs_d (V)"
  Demux4/1 -> Gain/1, Bus Creator/11  "Stator voltage Vs_q (V)"
  Park Transform1/1 -> Selector1/1
  nPolePairs/1 -> Hall sensor/1(thetae), Park Transform1/2, Park Transform/2
  wm/1 -> Bus Creator/21, Gain7/1  "Rotor speed wm (rad/s)"
  connections:
  PS-Simulink Converter1/LConn1 -- Line Voltage Sensor (Three-Phase)/RConn1
  PS-Simulink Converter/LConn1 -- Current Sensor/RConn1
  ~2/RConn1 -- Line Voltage Sensor (Three-Phase)/LConn1 -- Current Sensor/RConn2
  Current Sensor/LConn1 -- ~1/RConn1

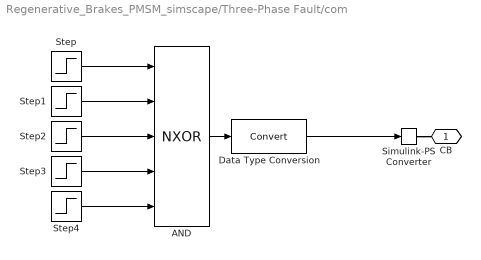
== system Regenerative_Brakes_PMSM_simscape/Three-Phase Fault/com ==
  AND : Logic  Operator=NXOR  Inputs=5  IconShape=distinctive  AllPortsSameDT=off  OutDataTypeStr=boolean
  Data Type Conversion : DataTypeConversion  SaturateOnIntegerOverflow=off  RndMeth=Floor
  Simulink-PS Converter : nesl_utility/Simulink-PS Converter  PhysicalDomain=network_engine_domain  SubClassName=ps_input  LeftPortType=input  RightPortType=output  PseudoPeriodic=off  Frequencies=[]  NoiseDistribution=none  NoiseParameters=[]  Unit=1  AffineConversion=off  FilteringAndDerivatives=provide  SimscapeFilterOrder=1  InputFilterTimeConstant=0.001  UdotUserProvided=0
  Step : Step  Time=Three_PhaseFault_class(0,[0.0166666666666667 0.0833333333333333],NaN,0.01,1000000,Inf,'on','off').objParamMappingDerived.NewDerivedParam.switchTime1  SampleTime=0
  Step1 : Step  Time=Three_PhaseFault_class(0,[0.0166666666666667 0.0833333333333333],NaN,0.01,1000000,Inf,'on','off').objParamMappingDerived.NewDerivedParam.switchTime2  SampleTime=0
  Step2 : Step  Time=Three_PhaseFault_class(0,[0.0166666666666667 0.0833333333333333],NaN,0.01,1000000,Inf,'on','off').objParamMappingDerived.NewDerivedParam.switchTime3  SampleTime=0
  Step3 : Step  Time=Three_PhaseFault_class(0,[0.0166666666666667 0.0833333333333333],NaN,0.01,1000000,Inf,'on','off').objParamMappingDerived.NewDerivedParam.switchTime4  SampleTime=0
  Step4 : Step  Time=Three_PhaseFault_class(0,[0.0166666666666667 0.0833333333333333],NaN,0.01,1000000,Inf,'on','off').objParamMappingDerived.NewDerivedParam.switchTime5  SampleTime=0
  CB : PMIOPort  Side=Right
  wires:
  Step2/1 -> AND/3
  Step/1 -> AND/1
  Step1/1 -> AND/2
  Step3/1 -> AND/4
  AND/1 -> Data Type Conversion/1
  Step4/1 -> AND/5
  Data Type Conversion/1 -> Simulink-PS Converter/1
  connections:
  Simulink-PS Converter/RConn1 -- CB/RConn1

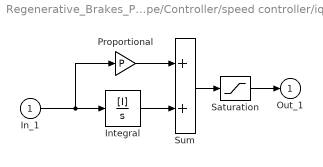
== system Regenerative_Brakes_PMSM_simscape/Controller/speed controller/iqref2 ==
  In_1 : Inport
  Integral : TransferFcn  Numerator=[I]  Denominator=[1 0]
  Proportional : Gain  Gain=P  SaturateOnIntegerOverflow=on  OutDataTypeStr=Inherit: Same as input  ParamDataTypeStr=Inherit: Same as input
  Saturation : Saturate  UpperLimit=max  LowerLimit=min
  Sum : Sum  InputSameDT=on  SaturateOnIntegerOverflow=on  OutDataTypeStr=Inherit: Same as first input
  Out_1 : Outport  InitialOutput=0  VectorParamsAs1DForOutWhenUnconnected=off
  wires:
  Integral/1 -> Sum/2
  In_1/1 -> Integral/1, Proportional/1
  Proportional/1 -> Sum/1
  Sum/1 -> Saturation/1
  Saturation/1 -> Out_1/1

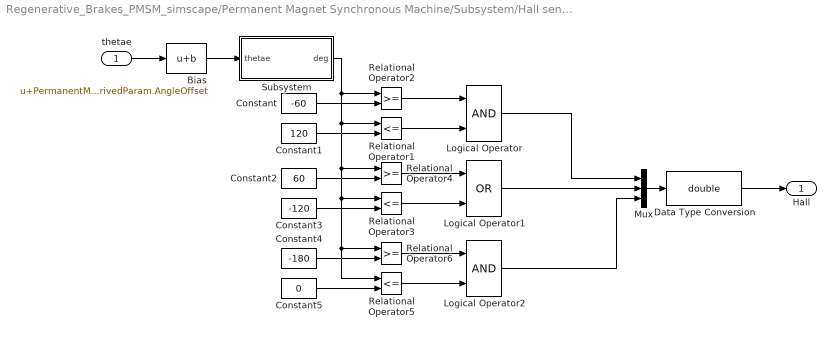
== system Regenerative_Brakes_PMSM_simscape/Permanent Magnet Synchronous Machine/Subsystem/Hall sensor ==
  thetae : Inport
  Bias : Bias  Bias=PermanentMagnetSynchrono_class('Torque Tm',[0.003334 0.000425 4 0],4,'Flux linkage established by magnets (V.s)',0.1821,132.1171,1.0926,'90 degrees behind phase A axis (modified Park)',[0 0 0 0],'Sinusoidal',120,'3',[0 0 0 0 0 0]).objParamMappingDerived.NewDerivedParam.AngleOffset  SaturateOnIntegerOverflow=off
  Constant : Constant  Value=-60
  Constant1 : Constant  Value=120
  Constant2 : Constant  Value=60
  Constant3 : Constant  Value=-120
  Constant4 : Constant  Value=-180
  Constant5 : Constant  Value=0
  Data Type Conversion : DataTypeConversion  OutDataTypeStr=double  SaturateOnIntegerOverflow=off  RndMeth=Floor
  Logical Operator : Logic  AllPortsSameDT=off  OutDataTypeStr=boolean
  Logical Operator1 : Logic  Operator=OR  AllPortsSameDT=off  OutDataTypeStr=boolean
  Logical Operator2 : Logic  AllPortsSameDT=off  OutDataTypeStr=boolean
  Mux : Mux  Inputs=3
  Relational Operator1 : RelationalOperator  Operator=<=
  Relational Operator2 : RelationalOperator
  Relational Operator3 : RelationalOperator  Operator=<=
  Relational Operator4 : RelationalOperator
  Relational Operator5 : RelationalOperator  Operator=<=
  Relational Operator6 : RelationalOperator
  Subsystem : Subsystem
  Hall : Outport  VectorParamsAs1DForOutWhenUnconnected=off
  wires:
  Bias/1 -> Subsystem/1(thetae)
  Data Type Conversion/1 -> Hall/1
  thetae/1 -> Bias/1
  Constant2/1 -> Relational Operator4/2
  Constant1/1 -> Relational Operator1/2
  Relational Operator4/1 -> Logical Operator1/1
  Constant/1 -> Relational Operator2/2
  Subsystem/1(deg) -> Relational Operator2/1, Relational Operator1/1, Relational Operator6/1, Relational Operator5/1, Relational Operator3/1, Relational Operator4/1
  Relational Operator1/1 -> Logical Operator/2
  Relational Operator2/1 -> Logical Operator/1
  Mux/1 -> Data Type Conversion/1
  Relational Operator3/1 -> Logical Operator1/2
  Constant5/1 -> Relational Operator5/2
  Constant4/1 -> Relational Operator6/2
  Relational Operator6/1 -> Logical Operator2/1
  Relational Operator5/1 -> Logical Operator2/2
  Logical Operator/1 -> Mux/1
  Logical Operator1/1 -> Mux/2
  Logical Operator2/1 -> Mux/3
  Constant3/1 -> Relational Operator3/2

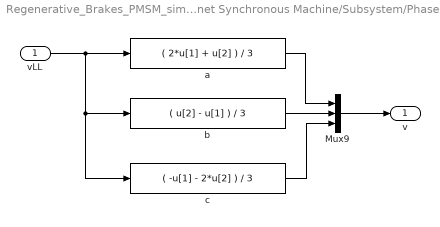
== system Regenerative_Brakes_PMSM_simscape/Permanent Magnet Synchronous Machine/Subsystem/Phase2neutral ==
  vLL : Inport
  Mux9 : Mux  Inputs=3
  a : Fcn  Expr=( 2*u[1] + u[2] ) / 3
  b : Fcn  Expr=( u[2] - u[1] ) / 3
  c : Fcn  Expr=( -u[1] - 2*u[2] ) / 3
  v : Outport
  wires:
  b/1 -> Mux9/2
  vLL/1 -> b/1, c/1, a/1
  c/1 -> Mux9/3
  a/1 -> Mux9/1
  Mux9/1 -> v/1

== system Regenerative_Brakes_PMSM_simscape/Permanent Magnet Synchronous Machine/Subsystem/Hall sensor/Subsystem ==
  thetae : Inport
  Trigonometric Function : Trigonometry  Operator=sincos
  Trigonometric Function2 : Trigonometry  Operator=atan2
  rad->deg : Gain  Gain=180/pi  SaturateOnIntegerOverflow=on  OutDataTypeStr=Inherit: Same as input  ParamDataTypeStr=Inherit: Same as input
  deg : Outport  VectorParamsAs1DForOutWhenUnconnected=off
  wires:
  thetae/1 -> Trigonometric Function/1
  Trigonometric Function/2 -> Trigonometric Function2/2
  rad->deg/1 -> deg/1
  Trigonometric Function/1 -> Trigonometric Function2/1
  Trigonometric Function2/1 -> rad->deg/1
